simulink model "MCC_Loop"  (Simulink 6.3)
settings: Solver=ode45  StartTime=0.0  StopTime=Inf  RelTol=1e-3
settings Model: LastModifiedBy=armigrs1

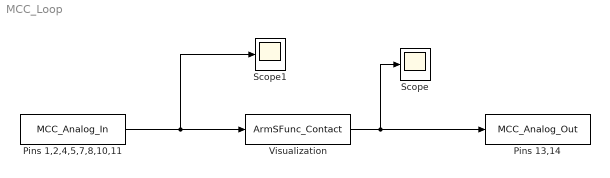
== system MCC_Loop ==
  Pins 1,2,4,5,7,8,10,11 : S-Function  FunctionName=MCC_Analog_In
  Pins 13,14 : S-Function  FunctionName=MCC_Analog_Out
  Scope : Scope
  Scope1 : Scope
  Visualization : S-Function  FunctionName=ArmSFunc_Contact
  wires:
  Pins 1,2,4,5,7,8,10,11/1 -> Visualization/1, Scope1/1
  Visualization/1 -> Scope/1, Pins 13,14/1
